simulink model "pwr_computeEnginePower"  (Simulink 7.3)
settings: Solver=FixedStepDiscrete  StartTime=0.0  StopTime=10.0  FixedStep=1  RelTol=1e-3
PostLoadFcn:
  | disp('Initialization script output/initEcBusObjects.m is run fom model callback PostLoadFcn')
  | run output/initEcBusObjects.m
libraries: simulink x14
settings Model: Creator=vranken  LastModifiedBy=vranken
settings DataIOCC: LimitDataPoints=off  SaveFormat=StructureWithTime
settings OptimizationCC: InlineParams=on  InlineInvariantSignals=on  ZeroExternalMemoryAtStartup=off  ZeroInternalMemoryAtStartup=off  EfficientFloat2IntCast=on  OptimizeModelRefInitCode=on  LifeSpan=1
settings DebuggingCC: SignalInfNanChecking=error  SignalRangeChecking=error  ReadBeforeWriteMsg=EnableAllAsError  WriteAfterWriteMsg=EnableAllAsError  WriteAfterReadMsg=EnableAllAsError  AlgebraicLoopMsg=error  ArtificialAlgebraicLoopMsg=error  CheckExecutionContextPreStartOutputMsg=on  CheckExecutionContextRuntimeOutputMsg=on  BlockPriorityViolationMsg=error  SolverPrmCheckMsg=error  InheritedTsInSrcMsg=none  DiscreteInheritContinuousMsg=error  SingleTaskRateTransMsg=error  SigSpecEnsureSampleTimeMsg=error  CheckMatrixSingularityMsg=error  IntegerOverflowMsg=error  ParameterUnderflowMsg=error  ParameterPrecisionLossMsg=none  ParameterTunabilityLossMsg=error  UnderSpecifiedDataTypeMsg=warning  UnnecessaryDatatypeConvMsg=warning  VectorMatrixConversionMsg=error  FcnCallInpInsideContextMsg=Enable All  SignalLabelMismatchMsg=warning  UnconnectedInputMsg=error  UnconnectedOutputMsg=error  UnconnectedLineMsg=error  SFcnCompatibilityMsg=warning  UniqueDataStoreMsg=warning  RootOutportRequireBusObject=error  ModelReferenceIOMsg=error  ModelReferenceIOMismatchMessage=error  ModelReferenceCSMismatchMessage=warning  UnknownTsInhSupMsg=error  ModelReferenceDataLoggingMessage=error  StrictBusMsg=ErrorOnBusTreatedAsVector
settings HardwareCC: ProdIntDivRoundTo=Zero  ProdEndianess=LittleEndian  ProdHWDeviceType=Intel->x86/Pentium  TargetIntDivRoundTo=Zero  TargetEndianess=LittleEndian  TargetHWDeviceType=Intel->x86/Pentium  ProdEqTarget=off
settings ModelReferenceCC: ModelReferenceNumInstancesAllowed=Single
settings RTWCC: SystemTargetFile=ert.tlc  GenCodeOnly=on  TemplateMakefile=ert_default_tmf  Description=Real-Time Workshop Embedded Coder  ProcessScript=ert_make_rtw_hook  RTWCompilerOptimization=On
settings CodeAppCC: ForceParamTrailComments=on  IgnoreCustomStorageClasses=off  MaxIdLength=64  CustomSymbolStrGlobalVar=pwr_$R$N$M  CustomSymbolStrType=pwr_$N$R$M_t  CustomSymbolStrMacro=PWR_$R$N$M
settings ERTTargetCC: TargetFunctionLibrary=C99 (ISO)  UtilityFuncGeneration=Shared location  MultiwordLength=2048  IncludeMdlTerminateFcn=off  SuppressErrorStatus=on  SupportAbsoluteTime=off  SupportNonFinite=off  SupportComplex=off  ParenthesesLevel=Minimum  InlinedParameterPlacement=NonHierarchical  ERTCustomFileTemplate=example_file_process.tlc

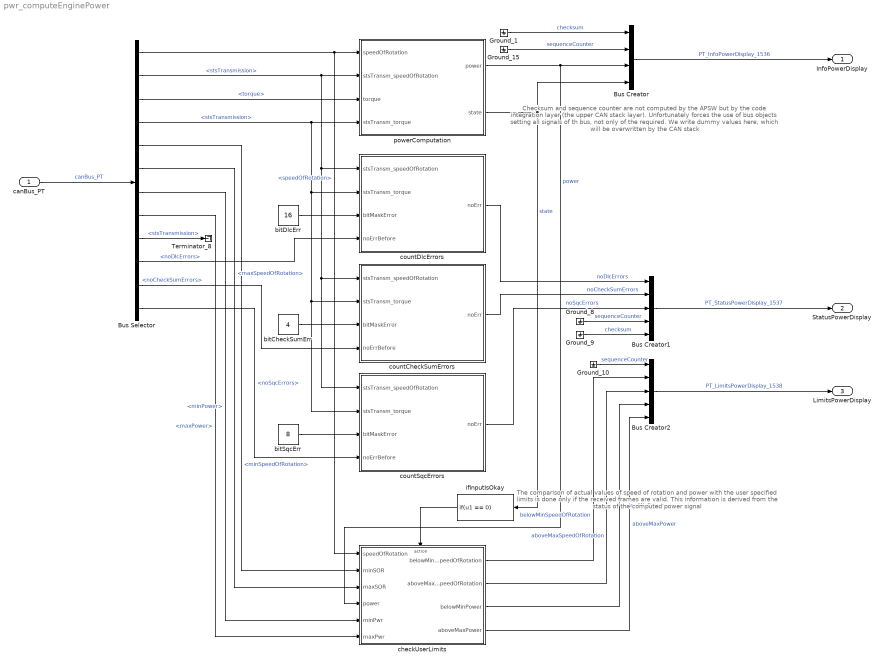
== system pwr_computeEnginePower ==
  note: The comparison of actual values of speed of rotation
      |  and power with the user specified limits is done only
      | if the received frames are valid. This information is
      | derived from the status of the computed power signal
  note: Checksum and sequence counter are not
      | computed by the APSW but by the code
      | integration layer (the upper CAN stack layer).
      | Unfortunately forces the use of bus objects
      | setting all signals of th bus, not only of
      | the required. We write dummy values here,
      | which will be overwritten by the CAN stack
  canBus_PT : Inport  UseBusObject=on  OutDataType=fixdt(1, 16)  OutScaling=2^0  BusOutputAsStruct=on
      settings: BusObject=cap_canBus_PT_t
  Bus Creator : BusCreator  UseBusObject=on  NonVirtualBus=on
      settings: BusObject=cap_PT_InfoPowerDisplay_1536_t
  Bus Creator1 : BusCreator  Inputs=5  UseBusObject=on  NonVirtualBus=on
      settings: BusObject=cap_PT_StatusPowerDisplay_1537_t
  Bus Creator2 : BusCreator  Inputs=5  UseBusObject=on  NonVirtualBus=on
      settings: BusObject=cap_PT_LimitsPowerDisplay_1538_t
  Bus Selector : BusSelector  OutputSignals=PT_StateEcu01_1024_sts.signals.speedOfRotation,PT_StateEcu01_1024_sts.stsTransmission,PT_StateEcu02_1040_sts.signals.torque,PT_StateEcu02_1040_sts.stsTransmission,PT_UserLimits_2032_sts.signals.minSpeedOfRotation,PT_UserLimits_2032_sts.signals.maxSpeedOfRotation,PT_UserLimits_2032_sts.signals.minPower,PT_UserLimits_2032_sts.signals.maxPower,PT_UserLimits_2032_sts.stsTransmission,PT_StatusPowerDisplay_1537_sts.signals.noDlcErrors,PT_StatusPowerDisplay_1537_sts.signals.noCheckSumErrors,PT_StatusPowerDisplay_1537_sts.signals.noSqcErrors
  Ground_{1,8..10,15} (5 alike) : Ground
  Terminator_8 : Terminator
  bitCheckSumErr : Constant  Value=4  OutDataTypeMode=uint8  OutDataType=fixdt(1, 16)  OutScaling=2^0  OutDataTypeStr=uint8
  bitDlcErr : Constant  Value=16  OutDataTypeMode=uint8  OutDataType=fixdt(1, 16)  OutScaling=2^0  OutDataTypeStr=uint8
  bitSqcErr : Constant  Value=8  OutDataTypeMode=uint8  OutDataType=fixdt(1, 16)  OutScaling=2^0  OutDataTypeStr=uint8
  checkUserLimits : Subsystem  TreatAsAtomicUnit=on  RTWFcnName=pwr_detectAndCountError
      settings: RTWFcnNameOpts=User specified
  countCheckSumErrors : Subsystem  TreatAsAtomicUnit=on  RTWFcnName=pwr_detectAndCountError
      settings: RTWFcnNameOpts=User specified
  countDlcErrors : Subsystem  TreatAsAtomicUnit=on  RTWFcnName=pwr_detectAndCountError
      settings: RTWFcnNameOpts=User specified
  countSqcErrors : Subsystem  TreatAsAtomicUnit=on  RTWFcnName=pwr_detectAndCountError
      settings: RTWFcnNameOpts=User specified
  ifInputIsOkay : If  IfExpression=u1 == 0  ShowElse=off
  powerComputation : Subsystem
  InfoPowerDisplay : Outport  UseBusObject=on  OutDataType=fixdt(1, 16)  OutScaling=2^0
      settings: BusObject=cap_PT_InfoPowerDisplay_1536_t
  StatusPowerDisplay : Outport  Port=2  UseBusObject=on  OutDataType=fixdt(1, 16)  OutScaling=2^0
      settings: BusObject=cap_PT_StatusPowerDisplay_1537_t
  LimitsPowerDisplay : Outport  Port=3  UseBusObject=on  OutDataType=fixdt(1, 16)  OutScaling=2^0
      settings: BusObject=cap_PT_LimitsPowerDisplay_1538_t
  wires:
  canBus_PT/1 -> Bus Selector/1  "canBus_PT"
  Bus Selector/1 -> powerComputation/1(speedOfRotation), checkUserLimits/1(speedOfRotation)  "<speedOfRotation>"
  Bus Selector/2 -> powerComputation/2(stsTransm_speedOfRotation), countDlcErrors/1(stsTransm_speedOfRotation), countCheckSumErrors/1(stsTransm_speedOfRotation), countSqcErrors/1(stsTransm_speedOfRotation)  "<stsTransmission>"
  Bus Creator/1 -> InfoPowerDisplay/1  "PT_InfoPowerDisplay_1536"
  Bus Creator1/1 -> StatusPowerDisplay/1  "PT_StatusPowerDisplay_1537"
  Bus Creator2/1 -> LimitsPowerDisplay/1  "PT_LimitsPowerDisplay_1538"
  Bus Selector/3 -> powerComputation/3(torque)  "<torque>"
  countDlcErrors/1(noErr) -> Bus Creator1/1  "noDlcErrors"
  countSqcErrors/1(noErr) -> Bus Creator1/3  "noSqcErrors"
  Ground_8/1 -> Bus Creator1/4  "sequenceCounter"
  Ground_9/1 -> Bus Creator1/5  "checksum"
  Ground_10/1 -> Bus Creator2/1  "sequenceCounter"
  checkUserLimits/1(belowMinSpeedOfRotation) -> Bus Creator2/2  "belowMinSpeedOfRotation"
  checkUserLimits/2(aboveMaxSpeedOfRotation) -> Bus Creator2/3  "aboveMaxSpeedOfRotation"
  checkUserLimits/3(belowMinPower) -> Bus Creator2/4  "belowMinPower"
  checkUserLimits/4(aboveMaxPower) -> Bus Creator2/5  "aboveMaxPower"
  Bus Selector/4 -> powerComputation/4(stsTransm_torque), countDlcErrors/2(stsTransm_torque), countCheckSumErrors/2(stsTransm_torque), countSqcErrors/2(stsTransm_torque)  "<stsTransmission>"
  Bus Selector/9 -> Terminator_8/1  "<stsTransmission>"
  Ground_1/1 -> Bus Creator/1  "checksum"
  Ground_15/1 -> Bus Creator/2  "sequenceCounter"
  powerComputation/1(power) -> Bus Creator/3, checkUserLimits/4(power)  "power"
  powerComputation/2(state) -> Bus Creator/4, ifInputIsOkay/1  "state"
  Bus Selector/11 -> countCheckSumErrors/4(noErrBefore)  "<noCheckSumErrors>"
  bitDlcErr/1 -> countDlcErrors/3(bitMaskError)
  bitCheckSumErr/1 -> countCheckSumErrors/3(bitMaskError)
  Bus Selector/10 -> countDlcErrors/4(noErrBefore)  "<noDlcErrors>"
  countCheckSumErrors/1(noErr) -> Bus Creator1/2  "noCheckSumErrors"
  bitSqcErr/1 -> countSqcErrors/3(bitMaskError)
  Bus Selector/12 -> countSqcErrors/4(noErrBefore)  "<noSqcErrors>"
  ifInputIsOkay/1 -> checkUserLimits/Action
  Bus Selector/5 -> checkUserLimits/2(minSOR)  "<minSpeedOfRotation>"
  Bus Selector/6 -> checkUserLimits/3(maxSOR)  "<maxSpeedOfRotation>"
  Bus Selector/7 -> checkUserLimits/5(minPwr)  "<minPower>"
  Bus Selector/8 -> checkUserLimits/6(maxPwr)  "<maxPower>"

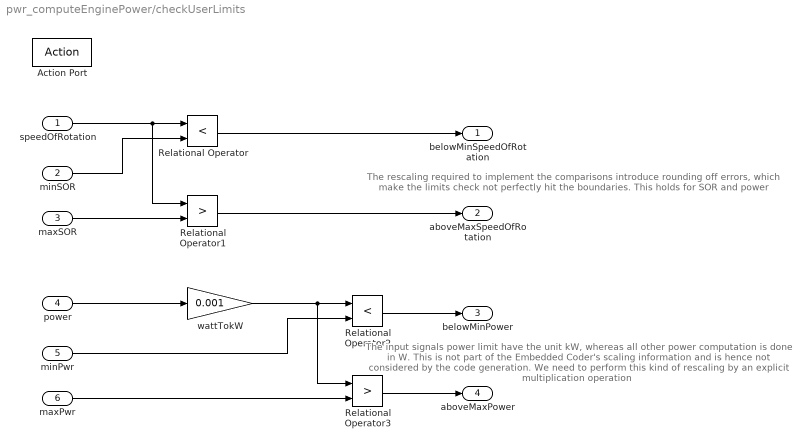
== system pwr_computeEnginePower/checkUserLimits ==
  note: The input signals power limit
      | have the unit kW, whereas all other
      | power computation is done in W.
      | This is not part of the Embedded
      | Coder's scaling information and is
      | hence not considered by the code
      | generation. We need to perform
      | this kind of rescaling by an explicit
      | multiplication operation
  note: The rescaling required to implement
      | the comparisons introduce rounding
      | off errors, which make the limits check
      | not perfectly hit the boundaries. This
      | holds for SOR and power
  speedOfRotation : Inport
  minSOR : Inport  Port=2
  maxSOR : Inport  Port=3
  power : Inport  Port=4
  minPwr : Inport  Port=5
  maxPwr : Inport  Port=6
  Action Port : ActionPort  ActionType=then
  Relational Operator : RelationalOperator  Operator=<  LogicOutDataTypeMode=boolean  LogicDataType=fixdt(0, 8)  OutDataTypeStr=boolean
  Relational Operator1 : RelationalOperator  Operator=>  LogicOutDataTypeMode=boolean  LogicDataType=fixdt(0, 8)  OutDataTypeStr=boolean
  Relational Operator2 : RelationalOperator  Operator=<  LogicOutDataTypeMode=boolean  LogicDataType=fixdt(0, 8)  OutDataTypeStr=boolean
  Relational Operator3 : RelationalOperator  Operator=>  LogicOutDataTypeMode=boolean  LogicDataType=fixdt(0, 8)  OutDataTypeStr=boolean
  wattTokW : Gain  Gain=0.001  ParameterDataType=fixdt(1, 16)  ParameterScaling=2^0  OutDataTypeMode=Specify via dialog  OutDataType=fixdt(0,16,2^-1,-10)  OutDataTypeStr=fixdt(0,16,2^-1,-10)
  belowMinSpeedOfRotation : Outport  OutDataType=fixdt(1, 16)  OutScaling=2^0
  aboveMaxSpeedOfRotation : Outport  Port=2  OutDataType=fixdt(1, 16)  OutScaling=2^0
  belowMinPower : Outport  Port=3  OutDataType=fixdt(1, 16)  OutScaling=2^0
  aboveMaxPower : Outport  Port=4  OutDataType=fixdt(1, 16)  OutScaling=2^0
  wires:
  speedOfRotation/1 -> Relational Operator/1, Relational Operator1/1
  minSOR/1 -> Relational Operator/2
  Relational Operator/1 -> belowMinSpeedOfRotation/1
  maxSOR/1 -> Relational Operator1/2
  Relational Operator1/1 -> aboveMaxSpeedOfRotation/1
  power/1 -> wattTokW/1
  minPwr/1 -> Relational Operator2/2
  Relational Operator2/1 -> belowMinPower/1
  maxPwr/1 -> Relational Operator3/2
  Relational Operator3/1 -> aboveMaxPower/1
  wattTokW/1 -> Relational Operator2/1, Relational Operator3/1

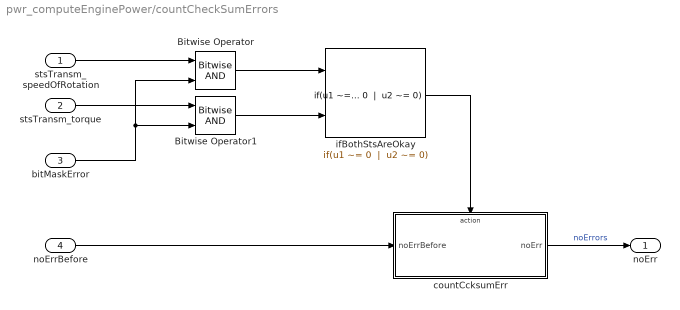
== system pwr_computeEnginePower/countCheckSumErrors ==
  stsTransm_speedOfRotation : Inport
  stsTransm_torque : Inport  Port=2
  bitMaskError : Inport  Port=3
  noErrBefore : Inport  Port=4
  Bitwise Operator : simulink/Logic and Bit Operations/Bitwise Operator  logicop=AND  UseBitMask=off  NumInputPorts=2  BitMask=bin2dec('11011001')  BitMaskRealWorld=Stored Integer
  Bitwise Operator1 : simulink/Logic and Bit Operations/Bitwise Operator  logicop=AND  UseBitMask=off  NumInputPorts=2  BitMask=bin2dec('11011001')  BitMaskRealWorld=Stored Integer
  countCcksumErr : Subsystem  TreatAsAtomicUnit=on
  ifBothStsAreOkay : If  NumInputs=2  IfExpression="u1 ~= 0  |  u2 ~= 0"  ShowElse=off
  noErr : Outport  OutDataType=fixdt(1, 16)  OutScaling=2^0
  wires:
  ifBothStsAreOkay/1 -> countCcksumErr/Action
  stsTransm_torque/1 -> Bitwise Operator1/1
  stsTransm_speedOfRotation/1 -> Bitwise Operator/1
  noErrBefore/1 -> countCcksumErr/1(noErrBefore)
  countCcksumErr/1(noErr) -> noErr/1  "noErrors"
  bitMaskError/1 -> Bitwise Operator/2, Bitwise Operator1/2
  Bitwise Operator/1 -> ifBothStsAreOkay/1
  Bitwise Operator1/1 -> ifBothStsAreOkay/2

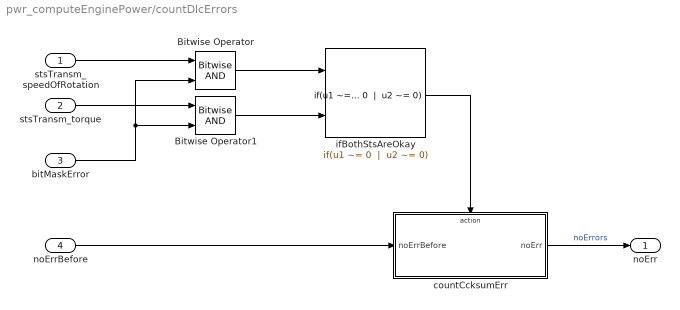
== system pwr_computeEnginePower/countDlcErrors ==
  stsTransm_speedOfRotation : Inport
  stsTransm_torque : Inport  Port=2
  bitMaskError : Inport  Port=3
  noErrBefore : Inport  Port=4
  Bitwise Operator : simulink/Logic and Bit Operations/Bitwise Operator  logicop=AND  UseBitMask=off  NumInputPorts=2  BitMask=bin2dec('11011001')  BitMaskRealWorld=Stored Integer
  Bitwise Operator1 : simulink/Logic and Bit Operations/Bitwise Operator  logicop=AND  UseBitMask=off  NumInputPorts=2  BitMask=bin2dec('11011001')  BitMaskRealWorld=Stored Integer
  countCcksumErr : Subsystem  TreatAsAtomicUnit=on
  ifBothStsAreOkay : If  NumInputs=2  IfExpression="u1 ~= 0  |  u2 ~= 0"  ShowElse=off
  noErr : Outport  OutDataType=fixdt(1, 16)  OutScaling=2^0
  wires:
  ifBothStsAreOkay/1 -> countCcksumErr/Action
  stsTransm_torque/1 -> Bitwise Operator1/1
  stsTransm_speedOfRotation/1 -> Bitwise Operator/1
  noErrBefore/1 -> countCcksumErr/1(noErrBefore)
  countCcksumErr/1(noErr) -> noErr/1  "noErrors"
  bitMaskError/1 -> Bitwise Operator/2, Bitwise Operator1/2
  Bitwise Operator/1 -> ifBothStsAreOkay/1
  Bitwise Operator1/1 -> ifBothStsAreOkay/2

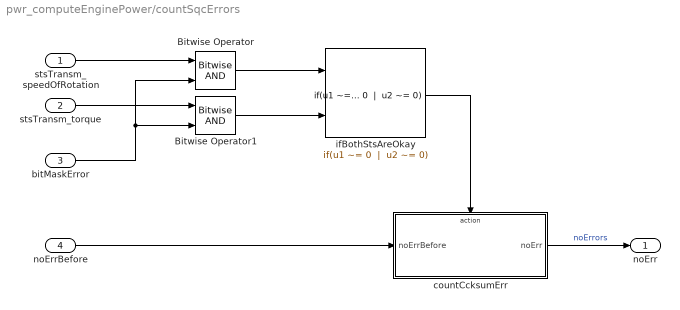
== system pwr_computeEnginePower/countSqcErrors ==
  stsTransm_speedOfRotation : Inport
  stsTransm_torque : Inport  Port=2
  bitMaskError : Inport  Port=3
  noErrBefore : Inport  Port=4
  Bitwise Operator : simulink/Logic and Bit Operations/Bitwise Operator  logicop=AND  UseBitMask=off  NumInputPorts=2  BitMask=bin2dec('11011001')  BitMaskRealWorld=Stored Integer
  Bitwise Operator1 : simulink/Logic and Bit Operations/Bitwise Operator  logicop=AND  UseBitMask=off  NumInputPorts=2  BitMask=bin2dec('11011001')  BitMaskRealWorld=Stored Integer
  countCcksumErr : Subsystem  TreatAsAtomicUnit=on
  ifBothStsAreOkay : If  NumInputs=2  IfExpression="u1 ~= 0  |  u2 ~= 0"  ShowElse=off
  noErr : Outport  OutDataType=fixdt(1, 16)  OutScaling=2^0
  wires:
  Bitwise Operator1/1 -> ifBothStsAreOkay/2
  Bitwise Operator/1 -> ifBothStsAreOkay/1
  bitMaskError/1 -> Bitwise Operator1/2, Bitwise Operator/2
  countCcksumErr/1(noErr) -> noErr/1  "noErrors"
  noErrBefore/1 -> countCcksumErr/1(noErrBefore)
  stsTransm_speedOfRotation/1 -> Bitwise Operator/1
  stsTransm_torque/1 -> Bitwise Operator1/1
  ifBothStsAreOkay/1 -> countCcksumErr/Action

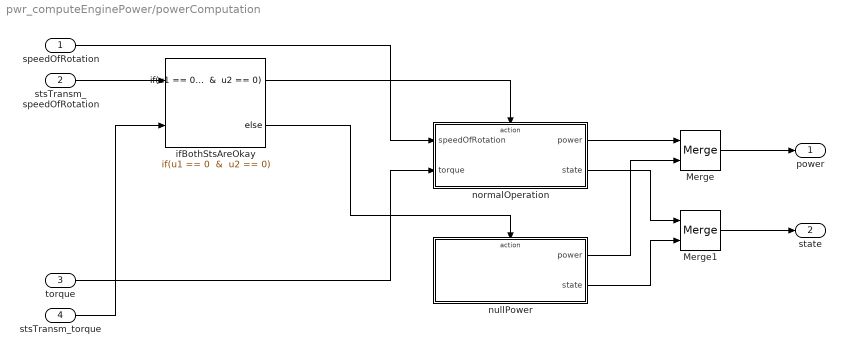
== system pwr_computeEnginePower/powerComputation ==
  speedOfRotation : Inport
  stsTransm_speedOfRotation : Inport  Port=2
  torque : Inport  Port=3
  stsTransm_torque : Inport  Port=4
  Merge : Merge
  Merge1 : Merge
  ifBothStsAreOkay : If  NumInputs=2  IfExpression="u1 == 0  &  u2 == 0"
  normalOperation : Subsystem  TreatAsAtomicUnit=on
  nullPower : Subsystem  TreatAsAtomicUnit=on
  power : Outport  OutDataType=fixdt(1, 16)  OutScaling=2^0
  state : Outport  Port=2  OutDataType=fixdt(1, 16)  OutScaling=2^0
  wires:
  speedOfRotation/1 -> normalOperation/1(speedOfRotation)
  stsTransm_speedOfRotation/1 -> ifBothStsAreOkay/1
  stsTransm_torque/1 -> ifBothStsAreOkay/2
  ifBothStsAreOkay/1 -> normalOperation/Action
  torque/1 -> normalOperation/2(torque)
  ifBothStsAreOkay/2 -> nullPower/Action
  normalOperation/1(power) -> Merge/1
  nullPower/1(power) -> Merge/2
  normalOperation/2(state) -> Merge1/1
  nullPower/2(state) -> Merge1/2
  Merge/1 -> power/1
  Merge1/1 -> state/1

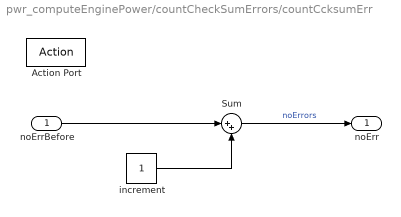
== system pwr_computeEnginePower/countCheckSumErrors/countCcksumErr ==
  noErrBefore : Inport
  Action Port : ActionPort  ActionType=then
  Sum : Sum  Inputs=|++  OutDataType=fixdt(1, 16)  OutScaling=2^0
  increment : Constant  OutDataTypeMode=uint8  OutDataType=fixdt(1, 16)  OutScaling=2^0  OutDataTypeStr=uint8
  noErr : Outport  OutDataType=fixdt(1, 16)  OutScaling=2^0
  wires:
  noErrBefore/1 -> Sum/1
  Sum/1 -> noErr/1  "noErrors"
  increment/1 -> Sum/2

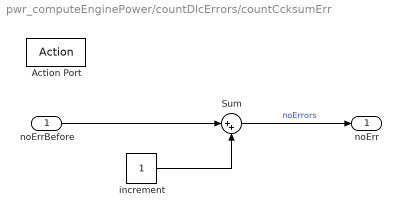
== system pwr_computeEnginePower/countDlcErrors/countCcksumErr ==
  noErrBefore : Inport
  Action Port : ActionPort  ActionType=then
  Sum : Sum  Inputs=|++  OutDataType=fixdt(1, 16)  OutScaling=2^0
  increment : Constant  OutDataTypeMode=uint8  OutDataType=fixdt(1, 16)  OutScaling=2^0  OutDataTypeStr=uint8
  noErr : Outport  OutDataType=fixdt(1, 16)  OutScaling=2^0
  wires:
  noErrBefore/1 -> Sum/1
  Sum/1 -> noErr/1  "noErrors"
  increment/1 -> Sum/2

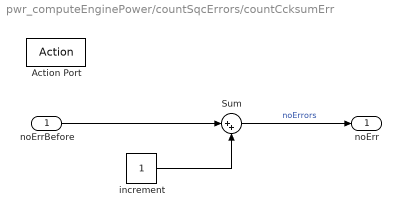
== system pwr_computeEnginePower/countSqcErrors/countCcksumErr ==
  noErrBefore : Inport
  Action Port : ActionPort  ActionType=then
  Sum : Sum  Inputs=|++  OutDataType=fixdt(1, 16)  OutScaling=2^0
  increment : Constant  OutDataTypeMode=uint8  OutDataType=fixdt(1, 16)  OutScaling=2^0  OutDataTypeStr=uint8
  noErr : Outport  OutDataType=fixdt(1, 16)  OutScaling=2^0
  wires:
  increment/1 -> Sum/2
  Sum/1 -> noErr/1  "noErrors"
  noErrBefore/1 -> Sum/1

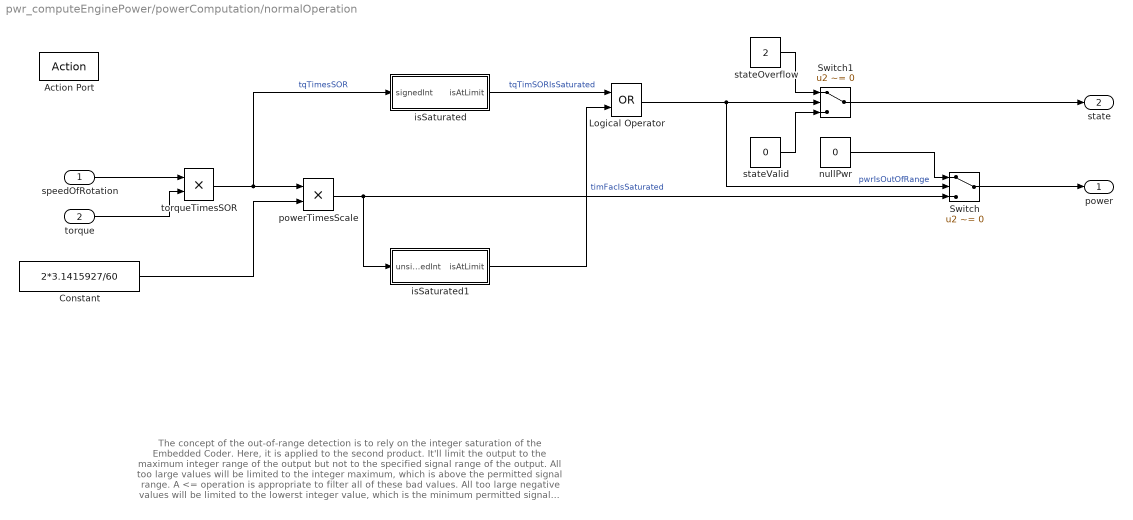
== system pwr_computeEnginePower/powerComputation/normalOperation ==
  note: The concept of the out-of-range detection is to rely on the integer saturation
      | of the Embedded Coder. Here, it is applied to the second product. It'll limit
      | the output to the maximum integer range of the output but not to the specified
      | signal range of the output.
      |   All too large values will be limited to the integer maximum, which is above
      | the permitted signal range. A <= operation is appropriate to filter all of these
      | bad values.
      |   All too large negative values will be limited to the lowerst integer value, which
      | is the minimum permitted signal value at the same time. It's a binary null. We
      | can't distinguish between a good but extreme value or a limited one if we see
      | the binary null. This is ignored; binary null is always considered a bad value.
      | Our logic effectively decreases the output signal range by one unit.
      |   A perfect out-of-range detection is nearly impossible in fixed point
      | computation since it requires some insight into the product operation. This
      | insight does the EC have during code generation but we don't have it on the
      | Simulink level.
      |  The best compromise would be the rule to never include the largest and
      | lowest integer values in the permitted signal range - then a safe detection
      | becomes possible in the way we present it here
  speedOfRotation : Inport
  torque : Inport  Port=2
  Action Port : ActionPort  ActionType=then
  Constant : Constant  Value=2*3.1415927/60  OutDataTypeMode=Specify via dialog  OutDataType=fixdt(0,16,19)  ConRadixGroup=Best Precision: Vector-wise  OutDataTypeStr=fixdt(0,16,19)
  Logical Operator : Logic  Operator=OR  AllPortsSameDT=off  OutDataTypeMode=boolean  LogicDataType=fixdt(0, 8)  OutDataTypeStr=boolean
  Switch : Switch  Criteria=u2 ~= 0  OutDataType=fixdt(1, 16)  OutScaling=2^0  OutDataTypeStr=Inherit: Inherit via back propagation
  Switch1 : Switch  Criteria=u2 ~= 0  OutDataType=fixdt(1, 16)  OutScaling=2^0  OutDataTypeStr=Inherit: Inherit via back propagation
  isSaturated : Subsystem
  isSaturated1 : Subsystem
  nullPwr : Constant  Value=0  OutDataType=fixdt(1, 16)  OutScaling=2^0  OutDataTypeStr=Inherit: Inherit via back propagation
  powerTimesScale : Product  OutDataTypeMode=Specify via dialog  OutDataType=fixdt(0,16,2^5,-500000)  OutDataTypeStr=fixdt(0,16,2^5,-500000)  RndMeth=Simplest  SaturateOnIntegerOverflow=on
  stateOverflow : Constant  Value=2  OutDataTypeMode=uint8  OutDataType=fixdt(1, 16)  OutScaling=2^0  OutDataTypeStr=uint8
  stateValid : Constant  Value=0  OutDataTypeMode=uint8  OutDataType=fixdt(1, 16)  OutScaling=2^0  OutDataTypeStr=uint8
  torqueTimesSOR : Product  OutMin=6553.5*(-500)  OutMax=6553.5*500  OutDataTypeMode=Specify via dialog  OutDataType=fixdt(1,32,9)  OutDataTypeStr=fixdt(1,32,9)  RndMeth=Simplest  SaturateOnIntegerOverflow=on
  power : Outport  OutDataType=fixdt(1, 16)  OutScaling=2^0  InitialOutput=0
  state : Outport  Port=2  OutDataType=fixdt(1, 16)  OutScaling=2^0  InitialOutput=1
  wires:
  speedOfRotation/1 -> torqueTimesSOR/1
  torque/1 -> torqueTimesSOR/2
  Constant/1 -> powerTimesScale/2
  powerTimesScale/1 -> isSaturated1/1(unsignedInt), Switch/3
  Switch/1 -> power/1
  Logical Operator/1 -> Switch1/2, Switch/2  "pwrIsOutOfRange"
  stateOverflow/1 -> Switch1/1
  stateValid/1 -> Switch1/3
  Switch1/1 -> state/1
  torqueTimesSOR/1 -> powerTimesScale/1, isSaturated/1(signedInt)  "tqTimesSOR"
  isSaturated/1(isAtLimit) -> Logical Operator/1  "tqTimSORIsSaturated"
  isSaturated1/1(isAtLimit) -> Logical Operator/2  "timFacIsSaturated"
  nullPwr/1 -> Switch/1

== system pwr_computeEnginePower/powerComputation/nullPower ==
  Action Port : ActionPort  ActionType=else
  Constant : Constant  Value=0  OutDataType=fixdt(1, 16)  OutScaling=2^0  OutDataTypeStr=Inherit: Inherit via back propagation
  stateInvalidInput : Constant  OutDataTypeMode=uint8  OutDataType=fixdt(1, 16)  OutScaling=2^0  OutDataTypeStr=uint8
  power : Outport  OutDataType=fixdt(1, 16)  OutScaling=2^0  InitialOutput=0
  state : Outport  Port=2  OutDataType=fixdt(1, 16)  OutScaling=2^0  InitialOutput=1
  wires:
  Constant/1 -> power/1
  stateInvalidInput/1 -> state/1

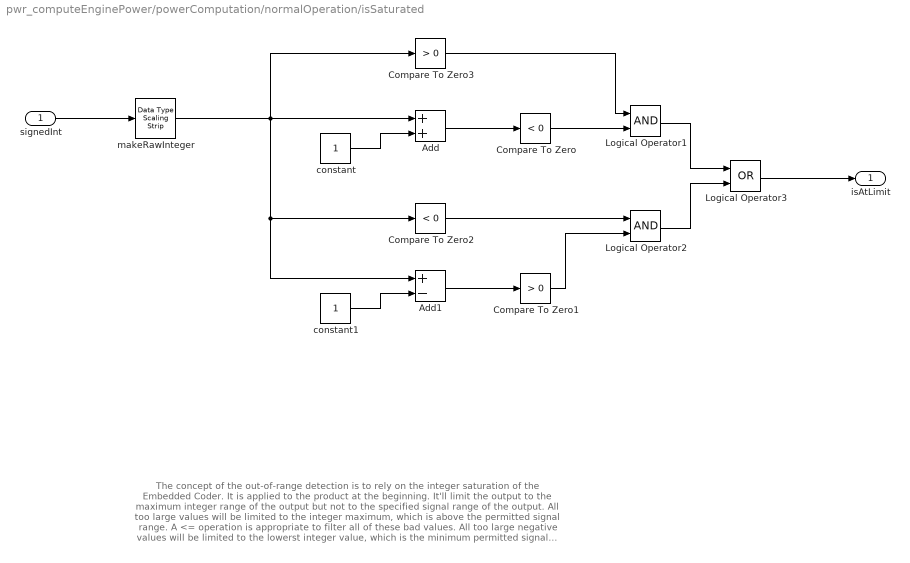
== system pwr_computeEnginePower/powerComputation/normalOperation/isSaturated ==
  note: The concept of the out-of-range detection is to rely on the integer saturation
      | of the Embedded Coder. It is applied to the product at the beginning. It'll limit
      | the output to the maximum integer range of the output but not to the specified
      | signal range of the output.
      |   All too large values will be limited to the integer maximum, which is above
      | the permitted signal range. A <= operation is appropriate to filter all of these
      | bad values.
      |   All too large negative values will be limited to the lowerst integer value, which
      | is the minimum permitted signal value at the same time. It's a binary null. We
      | can't distinguish between a good but extreme value or a limited one if we see
      | the binary null. This is ignored; binary null is always considered a bad value.
      | Our logic effectively decreases the output signal range by one unit.
      |   A perfect out-of-range detection is nearly impossible in fixed point
      | computation since it requires some insight into the product operation. This
      | insight does the EC have during code generation but we don't have it on the
      | Simulink level.
      |  The best compromise would be the rule to never include the largest and
      | lowest integer values in the permitted signal range - then a safe detection
      | becomes possible in the way we present it here
  signedInt : Inport
  Add : Sum  OutDataType=fixdt(1, 16)  OutScaling=2^-10  OutDataTypeStr=Inherit: Same as accumulator  RndMeth=Simplest
  Add1 : Sum  Inputs=+-  OutDataType=fixdt(1, 16)  OutScaling=2^-10  OutDataTypeStr=Inherit: Same as accumulator  RndMeth=Simplest
  Compare To Zero : simulink/Logic and Bit Operations/Compare To Zero  SystemSampleTime=-1  relop=<  LogicOutDataTypeMode=boolean  ZeroCross=off
  Compare To Zero1 : simulink/Logic and Bit Operations/Compare To Zero  SystemSampleTime=-1  relop=>  LogicOutDataTypeMode=boolean  ZeroCross=off
  Compare To Zero2 : simulink/Logic and Bit Operations/Compare To Zero  SystemSampleTime=-1  relop=<  LogicOutDataTypeMode=boolean  ZeroCross=off
  Compare To Zero3 : simulink/Logic and Bit Operations/Compare To Zero  SystemSampleTime=-1  relop=>  LogicOutDataTypeMode=boolean  ZeroCross=off
  Logical Operator1 : Logic  AllPortsSameDT=off  OutDataTypeMode=boolean  LogicDataType=fixdt(0, 8)  OutDataTypeStr=boolean
  Logical Operator2 : Logic  AllPortsSameDT=off  OutDataTypeMode=boolean  LogicDataType=fixdt(0, 8)  OutDataTypeStr=boolean
  Logical Operator3 : Logic  Operator=OR  AllPortsSameDT=off  OutDataTypeMode=boolean  LogicDataType=fixdt(0, 8)  OutDataTypeStr=boolean
  constant : Constant  OutDataType=fixdt(1, 16)  OutScaling=2^0  OutDataTypeStr=Inherit: Inherit via back propagation
  constant1 : Constant  OutDataType=fixdt(1, 16)  OutScaling=2^0  OutDataTypeStr=Inherit: Inherit via back propagation
  makeRawInteger : simulink/Signal Attributes/Data Type Scaling Strip  SystemSampleTime=-1
  isAtLimit : Outport
  wires:
  constant/1 -> Add/2
  signedInt/1 -> makeRawInteger/1
  Add/1 -> Compare To Zero/1
  constant1/1 -> Add1/2
  Add1/1 -> Compare To Zero1/1
  Compare To Zero2/1 -> Logical Operator2/1
  Compare To Zero1/1 -> Logical Operator2/2
  Compare To Zero3/1 -> Logical Operator1/1
  Compare To Zero/1 -> Logical Operator1/2
  Logical Operator1/1 -> Logical Operator3/1
  Logical Operator2/1 -> Logical Operator3/2
  Logical Operator3/1 -> isAtLimit/1
  makeRawInteger/1 -> Add/1, Add1/1, Compare To Zero2/1, Compare To Zero3/1

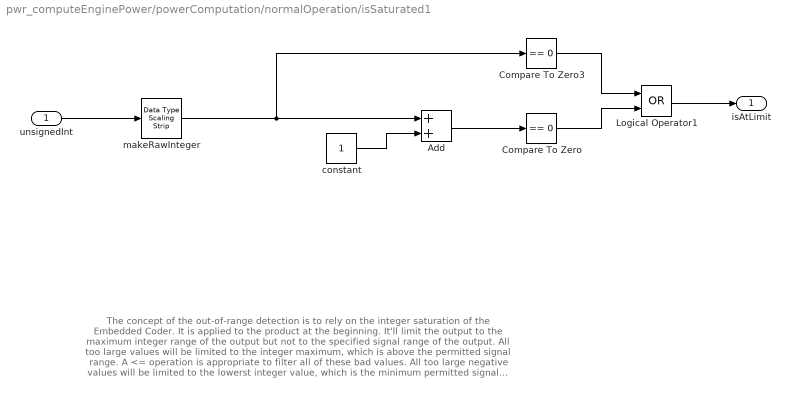
== system pwr_computeEnginePower/powerComputation/normalOperation/isSaturated1 ==
  note: The concept of the out-of-range detection is to rely on the integer saturation
      | of the Embedded Coder. It is applied to the product at the beginning. It'll limit
      | the output to the maximum integer range of the output but not to the specified
      | signal range of the output.
      |   All too large values will be limited to the integer maximum, which is above
      | the permitted signal range. A <= operation is appropriate to filter all of these
      | bad values.
      |   All too large negative values will be limited to the lowerst integer value, which
      | is the minimum permitted signal value at the same time. It's a binary null. We
      | can't distinguish between a good but extreme value or a limited one if we see
      | the binary null. This is ignored; binary null is always considered a bad value.
      | Our logic effectively decreases the output signal range by one unit.
      |   A perfect out-of-range detection is nearly impossible in fixed point
      | computation since it requires some insight into the product operation. This
      | insight does the EC have during code generation but we don't have it on the
      | Simulink level.
      |  The best compromise would be the rule to never include the largest and
      | lowest integer values in the permitted signal range - then a safe detection
      | becomes possible in the way we present it here
  unsignedInt : Inport
  Add : Sum  OutDataType=fixdt(1, 16)  OutScaling=2^-10  OutDataTypeStr=Inherit: Same as accumulator  RndMeth=Simplest
  Compare To Zero : simulink/Logic and Bit Operations/Compare To Zero  SystemSampleTime=-1  relop===  LogicOutDataTypeMode=boolean  ZeroCross=off
  Compare To Zero3 : simulink/Logic and Bit Operations/Compare To Zero  SystemSampleTime=-1  relop===  LogicOutDataTypeMode=boolean  ZeroCross=off
  Logical Operator1 : Logic  Operator=OR  AllPortsSameDT=off  OutDataTypeMode=boolean  LogicDataType=fixdt(0, 8)  OutDataTypeStr=boolean
  constant : Constant  OutDataType=fixdt(1, 16)  OutScaling=2^0  OutDataTypeStr=Inherit: Inherit via back propagation
  makeRawInteger : simulink/Signal Attributes/Data Type Scaling Strip  SystemSampleTime=-1
  isAtLimit : Outport
  wires:
  makeRawInteger/1 -> Compare To Zero3/1, Add/1
  Logical Operator1/1 -> isAtLimit/1
  Compare To Zero/1 -> Logical Operator1/2
  Compare To Zero3/1 -> Logical Operator1/1
  Add/1 -> Compare To Zero/1
  unsignedInt/1 -> makeRawInteger/1
  constant/1 -> Add/2
